simulink model "Model4"  (R2024b)
settings: Solver=VariableStepAuto  StartTime=0.0  StopTime=10.0  RelTol=1e-3
libraries: spsPower3phInstantaneousLib x8, spsThreePhaseParallelRLCLoadLib x4, spsThreePhaseVIMeasurementLib x4, spsThreePhaseBreakerLib x1, spsAsynchronousMachinepuUnitsLib x1, spsExcitationSystemLib x1, spsThreePhaseTransformerTwoWindingsLib x1, spsSynchronousMachinepuStandardLib x1, spsWindTurbineInductionGeneratorPhasorTypeLib x1, spspowerguiLib x1, sps_lib x1
settings Model: Creator=skill  LastModifiedBy=skill

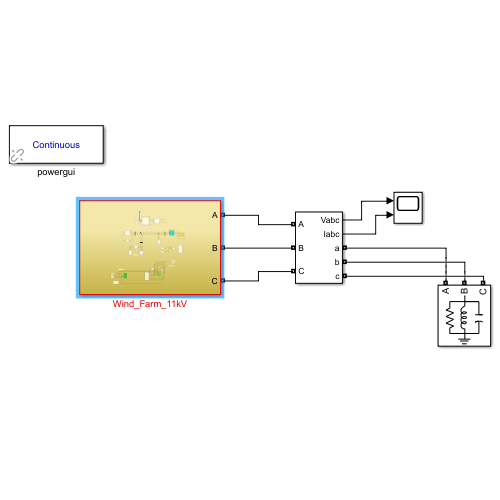
[thumbnail: Simulink's stored preview of the top-level diagram]
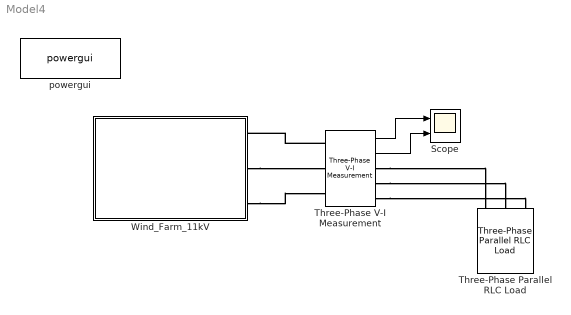
== system Model4 ==
  Scope : Scope  NumInputPorts=2
  Three-Phase Parallel RLC Load : spsThreePhaseParallelRLCLoadLib/Three-Phase Parallel RLC Load  LConnTagsString=A|B|C  Configuration=Y (grounded)  NominalVoltage=1000  Vabc=[1e3 1e3 1e3]  Vabcp=[1e3 1e3 1e3]  NominalFrequency=60  UnbalancedPower=off  ActivePower=10e3  InductivePower=100  CapacitivePower=100  Pabc=[10e3 9e3 11e3]  QLabc=[100 90 110]  QCabc=[100 90 110]  Pabcp=[10e3 9e3 11e3]  QLabcp=[100 90 110]  QCabcp=[100 90 110]  Measurements=None  LoadType=constant Z
  Three-Phase V-I Measurement : spsThreePhaseVIMeasurementLib/Three-Phase V-I Measurement  VoltageMeasurement=phase-to-ground  SetLabelV=off  LabelV=Vabc  Vpu=off  VpuLL=off  CurrentMeasurement=yes  SetLabelI=off  LabelI=Iabc  Ipu=off  Pbase=100e6  Vbase=500e3  OutputType=Complex  PhasorSimulation=off  PSBequivalent=0
  Wind_Farm_11kV : Subsystem
  powergui : sps_lib/powergui  Priority=1  SimulationMode=Continuous  SampleTime=50e-6  frequency=50  Iterations=50  frequencyindice=50  Pbase=100e6  ErrMax=1e-4  UnitsV=kV  UnitsW=MW  buscounter=0  FunctionMessages=off  echomessages=off  EnableUseOfTLC=off  CurrentSourceSwitches=off  DisableSnubberDevices=off  DisableRonSwitches=off  DisableVfSwitches=off  DisplayEquations=off  AutomaticDiscreteSolvers=off  SolverType=Tustin/Backward Euler (TBE)  Interpol=off  ExternalGateDelay=off  methode=off  Ts=100  x0status=blocks  SPID=on  SwTol=0  HookPort=off  NonlinearTolerance=1e-4  nMaxIteration=100  ContinueOnMaxIteration=off  RestoreLinks=warning  ResistiveCurrentMeasurement=off  Frange=[0:2:500]  Ylog=off  Xlog=on  ShowGrid=off  save=off  variable=ZData  structure=0  ZoomFFT=off  StartTime=0.0  cycles=1  DisplayStyle=1  fundamental=60  FreqAxis=off  MaxFrequency=1000  frequencyindicesteady=1  RmsSteady=1  display=off
  wires:
  Three-Phase V-I Measurement/1 -> Scope/1
  Three-Phase V-I Measurement/2 -> Scope/2
  connections:
  Three-Phase V-I Measurement/LConn1 -- Wind_Farm_11kV/RConn1
  Wind_Farm_11kV/RConn2 -- Three-Phase V-I Measurement/LConn2
  Wind_Farm_11kV/RConn3 -- Three-Phase V-I Measurement/LConn3
  Three-Phase V-I Measurement/RConn1 -- Three-Phase Parallel RLC Load/LConn1
  Three-Phase V-I Measurement/RConn2 -- Three-Phase Parallel RLC Load/LConn2
  Three-Phase V-I Measurement/RConn3 -- Three-Phase Parallel RLC Load/LConn3

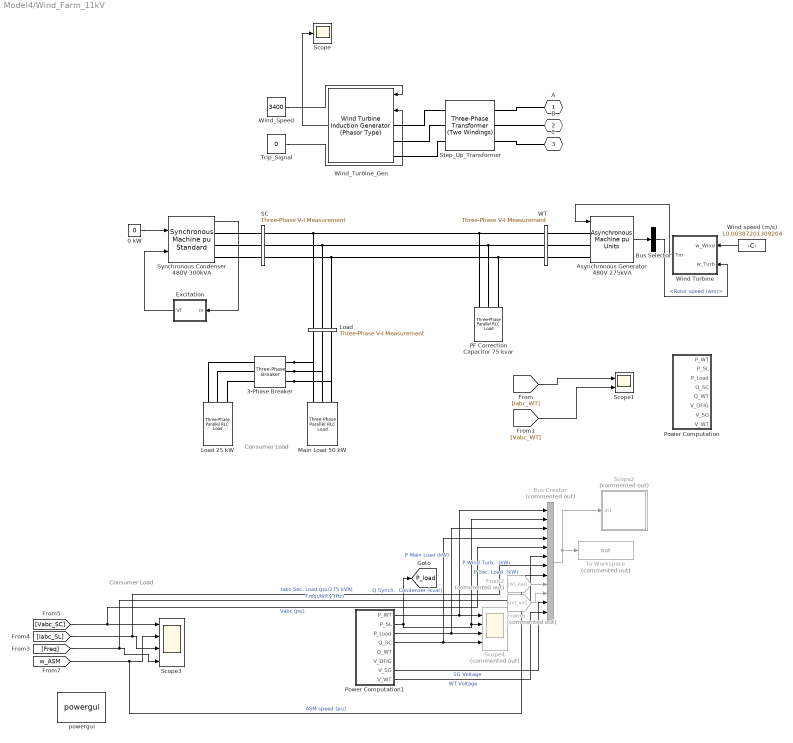
== system Model4/Wind_Farm_11kV ==
  note: Consumer Load
  note: Consumer Load
  0 kW : Constant  Value=0
  3-Phase Breaker : spsThreePhaseBreakerLib/Three-Phase Breaker  InitialState=open  SwitchA=on  SwitchB=on  SwitchC=on  SwitchTimes=[0.2]  External=off  BreakerResistance=0.001  SnubberResistance=1e6  SnubberCapacitance=inf  Measurements=None
      settings: AttributesFormatString=\n
  Asynchronous Generator 480V 275kVA : spsAsynchronousMachinepuUnitsLib/Asynchronous Machine pu Units  RotorType=Squirrel-cage  PresetModel=No  MechanicalLoad=Torque Tm  ShowDetailedParameters=on  ReferenceFrame=Rotor  Units=pu  MeasurementBus=off  NominalParameters=[ 275e3, 480, 60 ]  VoltageRatio=1  Stator=[ 0.016,0.06]  Rotor=[ 0.015,0.06]  Cage1=[0.01909 0.0397]  Cage2=[0.01909 0.0397]  Lm=3.5  Mechanical=[ 2,0,2 ]  PolePairs=2  InitialConditions=[-8.89496e-048 0 0.280896 0.280896 0.280896 -89.7425 150.258 30.2575]  SimulateSaturation=off  Saturation=[ 0 0 ; 0 0 ]  LoadFlowParameters=0  TsPowergui=0  TsBlock=-1  IterativeModel=Trapezoidal non iterative  IterativeDiscreteModel=Trapezoidal non iterative  Pmec=0
      settings: AttributesFormatString=\n
  Bus Creator : BusCreator  Commented=on  Inputs=12
  Bus Selector : BusSelector  OutputSignals=Mechanical.Rotor speed (wm)
  Excitation : Subsystem
  From2 : From  Commented=on  GotoTag=WT_Rea  TagVisibility=global
  From8 : From  Commented=on  GotoTag=rot_vol  TagVisibility=global
  Load : spsThreePhaseVIMeasurementLib/Three-Phase V-I Measurement  VoltageMeasurement=phase-to-ground  SetLabelV=on  LabelV=Vabc_Load  Vpu=on  VpuLL=off  CurrentMeasurement=yes  SetLabelI=on  LabelI=Iabc_Load  Ipu=on  Pbase=275e3  Vbase=480  OutputType=Magnitude  PhasorSimulation=off  PSBequivalent=0
  Load 25 kW : spsThreePhaseParallelRLCLoadLib/Three-Phase Parallel RLC Load  LConnTagsString=A|B|C  Configuration=Y (grounded)  NominalVoltage=480  Vabc=[1e3 1e3 1e3]  Vabcp=[1e3 1e3 1e3]  NominalFrequency=60  UnbalancedPower=off  ActivePower=25e3  InductivePower=0  CapacitivePower=0  Pabc=[10e3 9e3 11e3]  QLabc=[100 90 110]  QCabc=[100 90 110]  Pabcp=[10e3 9e3 11e3]  QLabcp=[100 90 110]  QCabcp=[100 90 110]  Measurements=None  LoadType=constant Z
  Main Load 50 kW : spsThreePhaseParallelRLCLoadLib/Three-Phase Parallel RLC Load  LConnTagsString=A|B|C  Configuration=Y (grounded)  NominalVoltage=480  Vabc=[1e3 1e3 1e3]  Vabcp=[1e3 1e3 1e3]  NominalFrequency=60  UnbalancedPower=off  ActivePower=50e3  InductivePower=0  CapacitivePower=0  Pabc=[10e3 9e3 11e3]  QLabc=[100 90 110]  QCabc=[100 90 110]  Pabcp=[10e3 9e3 11e3]  QLabcp=[100 90 110]  QCabcp=[100 90 110]  Measurements=None  LoadType=constant Z
  PF Correction Capacitor 75 kvar : spsThreePhaseParallelRLCLoadLib/Three-Phase Parallel RLC Load  LConnTagsString=A|B|C  Configuration=Delta  NominalVoltage=480  Vabc=[1e3 1e3 1e3]  Vabcp=[1e3 1e3 1e3]  NominalFrequency=60  UnbalancedPower=off  ActivePower=0  InductivePower=0  CapacitivePower=75e3  Pabc=[10e3 9e3 11e3]  QLabc=[100 90 110]  QCabc=[100 90 110]  Pabcp=[10e3 9e3 11e3]  QLabcp=[100 90 110]  QCabcp=[100 90 110]  Measurements=None  LoadType=constant Z
  Power Computation : Subsystem
  Power Computation1 : Subsystem
  SC : spsThreePhaseVIMeasurementLib/Three-Phase V-I Measurement  VoltageMeasurement=phase-to-ground  SetLabelV=on  LabelV=Vabc_SC  Vpu=on  VpuLL=off  CurrentMeasurement=yes  SetLabelI=on  LabelI=Iabc_SC  Ipu=on  Pbase=300e3  Vbase=480  OutputType=Magnitude  PhasorSimulation=off  PSBequivalent=0
  Scope : Scope
  Scope1 : Scope  NumInputPorts=2
  Scope2 : Subsystem  Commented=on
  Scope3 : Scope  NumInputPorts=4
  Scope4 : Scope  Commented=on  NumInputPorts=4
  Step_Up_Transformer : spsThreePhaseTransformerTwoWindingsLib/Three-Phase Transformer (Two Windings)  Winding1Connection=Yg  Winding2Connection=Yg  CoreType=Three single-phase transformers  SetSaturation=off  Hysteresis=off  DataFile='hysteresis'  SetInitialFlux=off  Measurements=None  UNITS=pu  NominalPower=[2e6, 50]  Winding1=[ 575 , 0.002 , 0.08 ]  Winding2=[ 11e3 , 0.002 , 0.08 ]  Rm=500  Lm=500  L0=0.5  Saturation=[ 0,0 ; 0.0024,1.2 ; 1.0,1.52 ]  InitialFluxes=[ 0.8 , -0.8 , 0.7 ]  BreakLoop=off  DiscreteSolver=Trapezoidal iterative  DataType=off  TransfoNumber=1
  Synchronous Condenser 480V 300kVA : spsSynchronousMachinepuStandardLib/Synchronous Machine pu Standard  PresetModel=No  MechanicalLoad=Mechanical power Pm  ShowDetailedParameters=on  RotorType=Salient-pole  Units=per unit standard parameters  MeasurementBus=off  NominalParameters=[ 300e3 480 60 ]  Reactances1=[ 3.23, 0.21, 0.15, 2.79, 1.03, 0.37, 0.09 ]  Reactances2=[2.24 0.17 0.12 1.02 0.13 0.08]  dAxisTimeConstants=Open-circuit  qAxisTimeConstants=Open-circuit  TimeConstants1="[ 4.4849  0.0681  0.1  ]"  TimeConstants2=[ 1.7, 0.008, 0.213, 0.004 ]  TimeConstants3="[  1.7 0.008 0.051266  ]"  TimeConstants4=[ 8.0, 0.03, 0.3371, 0.0295 ]  TimeConstants5="[ 0.08  0.019  0.004 ]"  TimeConstants6=[ 1.3201, 0.023, 1.0, 0.07 ]  TimeConstants7="[  0.08  0.019 0.051266  ]"  TimeConstants8=[ 1.3201, 0.0231, 0.3371, 0.0295 ]  StatorResistance=0.017  Mechanical=[ 1, 0, 2 ]  PolePairs=2  InitialConditions=[0 -89.2146 0.827 0.827 0.827 -86.4 153.6 33.6 2.71455]  SetSaturation=off  Saturation=[0.6404,0.7127,0.8441,0.9214,0.9956,1.082,1.19,1.316,1.457;0.7,0.7698,0.8872,0.9466,0.9969,1.046,1.1,1.151,1.201]  LoadFlowParameters=[2 0 0 0 0]  TsPowergui=0  TsBlock=-1  IterativeModel=Trapezoidal non iterative  IterativeDiscreteModel=Trapezoidal non iterative  BusType=PV  Pref=0  Qref=0  Qmin=-inf  Qmax=inf  PLF=0  QLF=0
  To Workspace : ToWorkspace  Commented=on  VariableName=out  SaveFormat=Timeseries  SampleTime=-1
  Trip_Signal : Constant  Value=0
  WT : spsThreePhaseVIMeasurementLib/Three-Phase V-I Measurement  VoltageMeasurement=phase-to-ground  SetLabelV=on  LabelV=Vabc_WT  Vpu=on  VpuLL=off  CurrentMeasurement=yes  SetLabelI=on  LabelI=Iabc_WT  Ipu=on  Pbase=275e3  Vbase=480  OutputType=Magnitude  PhasorSimulation=off  PSBequivalent=0
  Wind Turbine : Subsystem
  Wind speed (m/s) : Constant  Value=10.00387201309204
  Wind_Speed : Constant  Value=3400
  Wind_Turbine_Gen : spsWindTurbineInductionGeneratorPhasorTypeLib/Wind Turbine Induction Generator (Phasor Type)  ExternalTm=off  nom=[1.5e6/0.9, 575, 50]  sta=[ 0.004843, 0.1248]  rot=[ 0.004377, 0.1791]  Lm=6.77  mec=[5.04, 0.01, 3]  init="[ -0.01,0,   0,0,0,   0,0,0 ]"  pitch_angle=0  Pmec=1.5e6  wind_base=9  speed_nom=1  P_wind_base=1  K_pitch_gain=[5 25]  pitch_max=45  pitch_rate=2
      settings: LibrarySourceBlock=|
      | sps_lib/Electrical Machines/Wind Turbine
      | Induction Generator
      | (Phasor Type)
  powergui : spspowerguiLib/powergui  SimulationMode=Continuous  SampleTime=0  frequency=60  Iterations=50  frequencyindice=60  Pbase=100e6  ErrMax=1e-4  UnitsV=kV  UnitsW=MW  buscounter=0  FunctionMessages=off  echomessages=off  EnableUseOfTLC=off  CurrentSourceSwitches=on  DisableSnubberDevices=on  DisableRonSwitches=off  DisableVfSwitches=off  DisplayEquations=off  AutomaticDiscreteSolvers=off  SolverType=Tustin  Interpol=off  ExternalGateDelay=off  methode=off  Ts=0  x0status=blocks  SPID=off  SwTol=0  HookPort=off  NonlinearTolerance=1e-4  nMaxIteration=100  ContinueOnMaxIteration=off  RestoreLinks=warning  ResistiveCurrentMeasurement=off  Frange=[0:2:500]  Ylog=off  Xlog=on  ShowGrid=off  save=off  variable=ZData  structure=0  ZoomFFT=on  StartTime=0.0  cycles=1  DisplayStyle=1  fundamental=60  FreqAxis=off  MaxFrequency=1000  frequencyindicesteady=1  RmsSteady=1  display=off
  A : PMIOPort  Side=Right
  B : PMIOPort  Port=2  Side=Right
  C : PMIOPort  Port=3  Side=Right
  tag scope: P_load=global
  wires:
  Wind_Speed/1 -> Wind_Turbine_Gen/1
  Trip_Signal/1 -> Wind_Turbine_Gen/2
  Wind_Turbine_Gen/1 -> Scope/1
  Wind speed (m/s)/1 -> Wind Turbine/1(w_Wind)
  Asynchronous Generator 480V 275kVA/1 -> Bus Selector/1
  Bus Selector/1 -> Wind Turbine/2(w_Turb)  "<Rotor speed (wm)>"
  Wind Turbine/1(Tm) -> Asynchronous Generator 480V 275kVA/1
  Synchronous Condenser 480V 300kVA/1 -> Excitation/1(m)
  Excitation/1(Vf) -> Synchronous Condenser 480V 300kVA/2
  0 kW/1 -> Synchronous Condenser 480V 300kVA/1
  [Iabc_WT] -> Scope1/1
  [Vabc_WT] -> Scope1/2
  Power Computation1/1(P_WT) -> Bus Creator/1, Scope4/1  "P Wind Turb.  (kW)"
  Power Computation1/2(P_SL) -> Bus Creator/2, Scope4/2, [P_load]  "P Sec. Load  (kW)"
  Power Computation1/7(V_SG) -> Bus Creator/11  "SG Voltage"
  [Vabc_SC] -> Bus Creator/5, Scope3/1  "Vabc (pu)"
  Bus Creator/1 -> Scope2/1(In1), To Workspace/1
  [Iabc_SL] -> Bus Creator/7, Scope3/3  "Iabc Sec. Load (pu/275 kVA)"
  Power Computation1/3(P_Load) -> Bus Creator/3, Scope4/3  "P Main Load (kW)"
  Power Computation1/4(Q_SC) -> Bus Creator/4, Scope4/4  "Q Synch.  Condenser (kvar)"
  From8/1 -> Bus Creator/10
  [w_ASM] -> Bus Creator/8, Scope3/2  "ASM speed (pu)"
  From2/1 -> Bus Creator/9
  [Freq] -> Bus Creator/6, Scope3/4  "Frequency (Hz)"
  Power Computation1/8(V_WT) -> Bus Creator/12  "WT Voltage"
  connections:
  Wind_Turbine_Gen/LConn1 -- Step_Up_Transformer/LConn1
  Wind_Turbine_Gen/LConn2 -- Step_Up_Transformer/LConn2
  Wind_Turbine_Gen/LConn3 -- Step_Up_Transformer/LConn3
  Step_Up_Transformer/RConn1 -- A/RConn1
  Step_Up_Transformer/RConn2 -- B/RConn1
  Step_Up_Transformer/RConn3 -- C/RConn1
  WT/RConn1 -- Asynchronous Generator 480V 275kVA/LConn1
  WT/RConn2 -- Asynchronous Generator 480V 275kVA/LConn2
  WT/RConn3 -- Asynchronous Generator 480V 275kVA/LConn3
  SC/RConn1 -- Load/LConn1 -- PF Correction Capacitor 75 kvar/LConn1 -- WT/LConn1
  SC/RConn2 -- Load/LConn2 -- WT/LConn2 -- PF Correction Capacitor 75 kvar/LConn2
  SC/RConn3 -- Load/LConn3 -- PF Correction Capacitor 75 kvar/LConn3 -- WT/LConn3
  Synchronous Condenser 480V 300kVA/RConn1 -- SC/LConn1
  Synchronous Condenser 480V 300kVA/RConn2 -- SC/LConn2
  Synchronous Condenser 480V 300kVA/RConn3 -- SC/LConn3
  3-Phase Breaker/LConn2 -- Load/RConn2 -- Main Load 50 kW/LConn2
  3-Phase Breaker/LConn1 -- Load/RConn1 -- Main Load 50 kW/LConn1
  3-Phase Breaker/LConn3 -- Load/RConn3 -- Main Load 50 kW/LConn3
  3-Phase Breaker/RConn2 -- Load 25 kW/LConn2
  3-Phase Breaker/RConn1 -- Load 25 kW/LConn1
  3-Phase Breaker/RConn3 -- Load 25 kW/LConn3

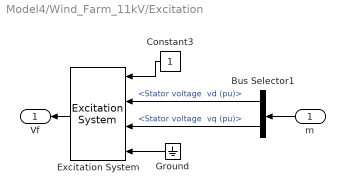
== system Model4/Wind_Farm_11kV/Excitation ==
  m : Inport
  Bus Selector1 : BusSelector  OutputSignals="dq0 components.Stator voltage  vd (pu),dq0 components.Stator voltage  vq (pu)"
  Constant3 : Constant
  Excitation System : spsExcitationSystemLib/Excitation System  tr=20e-3  reg=[ 300, 0.001 ]  exc=[ 1, 0 ]  tgr=[ 0, 0 ]  damp=[ 0.001, 0.1 ]  sat=[ 0, 0 ]  lim=[ -11.5, 11.5, 0 ]  v0=[1,2.71455]
  Ground : Ground
  Vf : Outport  VectorParamsAs1DForOutWhenUnconnected=off
  wires:
  Constant3/1 -> Excitation System/1
  Ground/1 -> Excitation System/4
  m/1 -> Bus Selector1/1
  Excitation System/1 -> Vf/1
  Bus Selector1/1 -> Excitation System/2  "<Stator voltage  vd (pu)>"
  Bus Selector1/2 -> Excitation System/3  "<Stator voltage  vq (pu)>"

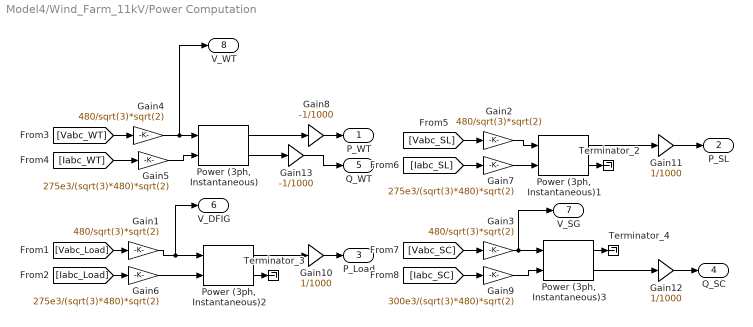
== system Model4/Wind_Farm_11kV/Power Computation ==
  Gain{1..4} (4 alike) : Gain  Gain=480/sqrt(3)*sqrt(2)  SaturateOnIntegerOverflow=on  OutDataTypeStr=Inherit: Same as input  ParamDataTypeStr=Inherit: Same as input
  Gain10 : Gain  Gain=1/1000  SaturateOnIntegerOverflow=on  OutDataTypeStr=Inherit: Same as input  ParamDataTypeStr=Inherit: Same as input
  Gain11 : Gain  Gain=1/1000  SaturateOnIntegerOverflow=on  OutDataTypeStr=Inherit: Same as input  ParamDataTypeStr=Inherit: Same as input
  Gain12 : Gain  Gain=1/1000  SaturateOnIntegerOverflow=on  OutDataTypeStr=Inherit: Same as input  ParamDataTypeStr=Inherit: Same as input
  Gain13 : Gain  Gain=-1/1000  SaturateOnIntegerOverflow=on  OutDataTypeStr=Inherit: Same as input  ParamDataTypeStr=Inherit: Same as input
  Gain5 : Gain  Gain=275e3/(sqrt(3)*480)*sqrt(2)  SaturateOnIntegerOverflow=on  OutDataTypeStr=Inherit: Same as input  ParamDataTypeStr=Inherit: Same as input
  Gain6 : Gain  Gain=275e3/(sqrt(3)*480)*sqrt(2)  SaturateOnIntegerOverflow=on  OutDataTypeStr=Inherit: Same as input  ParamDataTypeStr=Inherit: Same as input
  Gain7 : Gain  Gain=275e3/(sqrt(3)*480)*sqrt(2)  SaturateOnIntegerOverflow=on  OutDataTypeStr=Inherit: Same as input  ParamDataTypeStr=Inherit: Same as input
  Gain8 : Gain  Gain=-1/1000  SaturateOnIntegerOverflow=on  OutDataTypeStr=Inherit: Same as input  ParamDataTypeStr=Inherit: Same as input
  Gain9 : Gain  Gain=300e3/(sqrt(3)*480)*sqrt(2)  SaturateOnIntegerOverflow=on  OutDataTypeStr=Inherit: Same as input  ParamDataTypeStr=Inherit: Same as input
  Power (3ph, Instantaneous){,1..3} (4 alike) : spsPower3phInstantaneousLib/Power (3ph, Instantaneous)
  Terminator_2 : Terminator
  Terminator_3 : Terminator
  Terminator_4 : Terminator
  P_WT : Outport  VectorParamsAs1DForOutWhenUnconnected=off
  P_SL : Outport  Port=2  VectorParamsAs1DForOutWhenUnconnected=off
  P_Load : Outport  Port=3  VectorParamsAs1DForOutWhenUnconnected=off
  Q_SC : Outport  Port=4  VectorParamsAs1DForOutWhenUnconnected=off
  Q_WT : Outport  Port=5  VectorParamsAs1DForOutWhenUnconnected=off
  V_DFIG : Outport  Port=6  VectorParamsAs1DForOutWhenUnconnected=off
  V_SG : Outport  Port=7  VectorParamsAs1DForOutWhenUnconnected=off
  V_WT : Outport  Port=8  VectorParamsAs1DForOutWhenUnconnected=off
  wires:
  "Power (3ph, Instantaneous)1"/1 -> Gain11/1
  [Vabc_WT] -> Gain4/1
  [Iabc_WT] -> Gain5/1
  Gain4/1 -> V_WT/1, "Power (3ph, Instantaneous)"/1
  Gain5/1 -> "Power (3ph, Instantaneous)"/2
  [Vabc_Load] -> Gain1/1
  [Iabc_Load] -> Gain6/1
  Gain1/1 -> V_DFIG/1, "Power (3ph, Instantaneous)2"/1
  Gain6/1 -> "Power (3ph, Instantaneous)2"/2
  [Vabc_SL] -> Gain2/1
  [Iabc_SL] -> Gain7/1
  Gain2/1 -> "Power (3ph, Instantaneous)1"/1
  Gain7/1 -> "Power (3ph, Instantaneous)1"/2
  "Power (3ph, Instantaneous)2"/1 -> Gain10/1
  "Power (3ph, Instantaneous)"/1 -> Gain8/1
  Gain8/1 -> P_WT/1
  "Power (3ph, Instantaneous)3"/2 -> Gain12/1
  [Vabc_SC] -> Gain3/1
  [Iabc_SC] -> Gain9/1
  Gain3/1 -> V_SG/1, "Power (3ph, Instantaneous)3"/1
  Gain9/1 -> "Power (3ph, Instantaneous)3"/2
  Gain10/1 -> P_Load/1
  Gain11/1 -> P_SL/1
  Gain12/1 -> Q_SC/1
  "Power (3ph, Instantaneous)"/2 -> Gain13/1
  "Power (3ph, Instantaneous)1"/2 -> Terminator_2/1
  "Power (3ph, Instantaneous)2"/2 -> Terminator_3/1
  "Power (3ph, Instantaneous)3"/1 -> Terminator_4/1
  Gain13/1 -> Q_WT/1

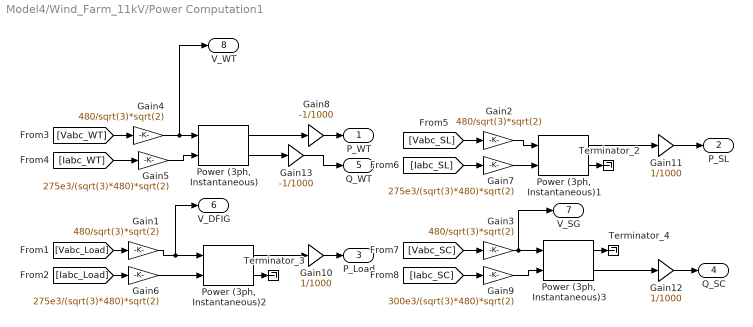
== system Model4/Wind_Farm_11kV/Power Computation1 ==
  Gain{1..4} (4 alike) : Gain  Gain=480/sqrt(3)*sqrt(2)  SaturateOnIntegerOverflow=on  OutDataTypeStr=Inherit: Same as input  ParamDataTypeStr=Inherit: Same as input
  Gain10 : Gain  Gain=1/1000  SaturateOnIntegerOverflow=on  OutDataTypeStr=Inherit: Same as input  ParamDataTypeStr=Inherit: Same as input
  Gain11 : Gain  Gain=1/1000  SaturateOnIntegerOverflow=on  OutDataTypeStr=Inherit: Same as input  ParamDataTypeStr=Inherit: Same as input
  Gain12 : Gain  Gain=1/1000  SaturateOnIntegerOverflow=on  OutDataTypeStr=Inherit: Same as input  ParamDataTypeStr=Inherit: Same as input
  Gain13 : Gain  Gain=-1/1000  SaturateOnIntegerOverflow=on  OutDataTypeStr=Inherit: Same as input  ParamDataTypeStr=Inherit: Same as input
  Gain5 : Gain  Gain=275e3/(sqrt(3)*480)*sqrt(2)  SaturateOnIntegerOverflow=on  OutDataTypeStr=Inherit: Same as input  ParamDataTypeStr=Inherit: Same as input
  Gain6 : Gain  Gain=275e3/(sqrt(3)*480)*sqrt(2)  SaturateOnIntegerOverflow=on  OutDataTypeStr=Inherit: Same as input  ParamDataTypeStr=Inherit: Same as input
  Gain7 : Gain  Gain=275e3/(sqrt(3)*480)*sqrt(2)  SaturateOnIntegerOverflow=on  OutDataTypeStr=Inherit: Same as input  ParamDataTypeStr=Inherit: Same as input
  Gain8 : Gain  Gain=-1/1000  SaturateOnIntegerOverflow=on  OutDataTypeStr=Inherit: Same as input  ParamDataTypeStr=Inherit: Same as input
  Gain9 : Gain  Gain=300e3/(sqrt(3)*480)*sqrt(2)  SaturateOnIntegerOverflow=on  OutDataTypeStr=Inherit: Same as input  ParamDataTypeStr=Inherit: Same as input
  Power (3ph, Instantaneous){,1..3} (4 alike) : spsPower3phInstantaneousLib/Power (3ph, Instantaneous)
  Terminator_2 : Terminator
  Terminator_3 : Terminator
  Terminator_4 : Terminator
  P_WT : Outport  VectorParamsAs1DForOutWhenUnconnected=off
  P_SL : Outport  Port=2  VectorParamsAs1DForOutWhenUnconnected=off
  P_Load : Outport  Port=3  VectorParamsAs1DForOutWhenUnconnected=off
  Q_SC : Outport  Port=4  VectorParamsAs1DForOutWhenUnconnected=off
  Q_WT : Outport  Port=5  VectorParamsAs1DForOutWhenUnconnected=off
  V_DFIG : Outport  Port=6  VectorParamsAs1DForOutWhenUnconnected=off
  V_SG : Outport  Port=7  VectorParamsAs1DForOutWhenUnconnected=off
  V_WT : Outport  Port=8  VectorParamsAs1DForOutWhenUnconnected=off
  wires:
  "Power (3ph, Instantaneous)1"/1 -> Gain11/1
  [Vabc_WT] -> Gain4/1
  [Iabc_WT] -> Gain5/1
  Gain4/1 -> V_WT/1, "Power (3ph, Instantaneous)"/1
  Gain5/1 -> "Power (3ph, Instantaneous)"/2
  [Vabc_Load] -> Gain1/1
  [Iabc_Load] -> Gain6/1
  Gain1/1 -> V_DFIG/1, "Power (3ph, Instantaneous)2"/1
  Gain6/1 -> "Power (3ph, Instantaneous)2"/2
  [Vabc_SL] -> Gain2/1
  [Iabc_SL] -> Gain7/1
  Gain2/1 -> "Power (3ph, Instantaneous)1"/1
  Gain7/1 -> "Power (3ph, Instantaneous)1"/2
  "Power (3ph, Instantaneous)2"/1 -> Gain10/1
  "Power (3ph, Instantaneous)"/1 -> Gain8/1
  Gain8/1 -> P_WT/1
  "Power (3ph, Instantaneous)3"/2 -> Gain12/1
  [Vabc_SC] -> Gain3/1
  [Iabc_SC] -> Gain9/1
  Gain3/1 -> V_SG/1, "Power (3ph, Instantaneous)3"/1
  Gain9/1 -> "Power (3ph, Instantaneous)3"/2
  Gain10/1 -> P_Load/1
  Gain11/1 -> P_SL/1
  Gain12/1 -> Q_SC/1
  "Power (3ph, Instantaneous)"/2 -> Gain13/1
  "Power (3ph, Instantaneous)1"/2 -> Terminator_2/1
  "Power (3ph, Instantaneous)2"/2 -> Terminator_3/1
  "Power (3ph, Instantaneous)3"/1 -> Terminator_4/1
  Gain13/1 -> Q_WT/1

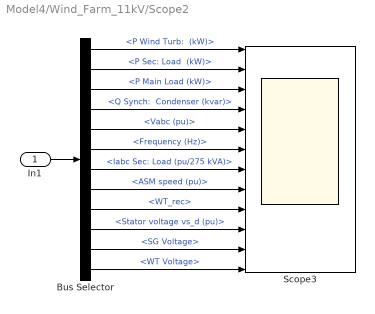
== system Model4/Wind_Farm_11kV/Scope2 ==
  In1 : Inport
  Bus Selector : BusSelector  OutputSignals="P Wind Turb:  (kW),P Sec: Load  (kW),P Main Load (kW),Q Synch:  Condenser (kvar),Vabc (pu),Frequency (Hz),Iabc Sec: Load (pu/275 kVA),ASM speed (pu),WT_rec,Stator voltage vs_d (pu),SG Voltage,WT Voltage"
  Scope3 : Scope  NumInputPorts=12
  wires:
  In1/1 -> Bus Selector/1
  Bus Selector/1 -> Scope3/1  "<P Wind Turb:  (kW)>"
  Bus Selector/2 -> Scope3/2  "<P Sec: Load  (kW)>"
  Bus Selector/3 -> Scope3/3  "<P Main Load (kW)>"
  Bus Selector/4 -> Scope3/4  "<Q Synch:  Condenser (kvar)>"
  Bus Selector/5 -> Scope3/5  "<Vabc (pu)>"
  Bus Selector/6 -> Scope3/6  "<Frequency (Hz)>"
  Bus Selector/7 -> Scope3/7  "<Iabc Sec: Load (pu/275 kVA)>"
  Bus Selector/8 -> Scope3/8  "<ASM speed (pu)>"
  Bus Selector/9 -> Scope3/9  "<WT_rec>"
  Bus Selector/10 -> Scope3/10  "<Stator voltage vs_d (pu)>"
  Bus Selector/11 -> Scope3/11  "<SG Voltage>"
  Bus Selector/12 -> Scope3/12  "<WT Voltage>"

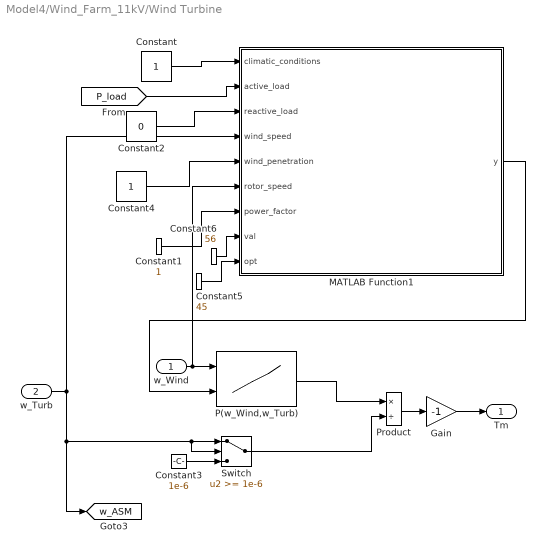
== system Model4/Wind_Farm_11kV/Wind Turbine ==
  w_Wind : Inport
  w_Turb : Inport  Port=2
  Constant : Constant
  Constant1 : Constant
  Constant2 : Constant  Value=0
  Constant3 : Constant  Value=1e-6
  Constant4 : Constant
  Constant5 : Constant  Value=45
  Constant6 : Constant  Value=56
  Gain : Gain  Gain=-1  SaturateOnIntegerOverflow=on  OutDataTypeStr=Inherit: Same as input  ParamDataTypeStr=Inherit: Same as input
  MATLAB Function1 : MATLAB Function  TreatAsAtomicUnit=on
  P(w_Wind,w_Turb) : Lookup_n-D  BreakpointsForDimension1=[0 5 6 7 8 9 10 11 12]  BreakpointsForDimension2=[0 571.55 685.8 800.15 914.4 1028.8 1143.1 1257.4 1371.7 1486 1600.3 1714.6 1828.9 1943.2 2057.5 2171.8 2286.1 2400.5 2514.7 2629.1 2743.3 2857.7 2971.9 3086.3 3200.5 3314.9 3429.2]  Table=[0 5 6 7 8 9 10 11 12]  InternalRulePriority=Speed  RndMeth=Simplest
      settings: InputPortMap=u0,u1
  Product : Product  Inputs=*/  InputSameDT=on  SaturateOnIntegerOverflow=on  OutDataTypeStr=Inherit: Same as first input
  Switch : Switch  Threshold=1e-6
  Tm : Outport  VectorParamsAs1DForOutWhenUnconnected=off
  tag scope: w_ASM=global
  wires:
  Constant3/1 -> Switch/3
  w_Wind/1 -> MATLAB Function1/6(rotor_speed), P(w_Wind,w_Turb)/1
  P(w_Wind,w_Turb)/1 -> Product/1
  Switch/1 -> Product/2
  Product/1 -> Gain/1
  Gain/1 -> Tm/1
  [P_load] -> MATLAB Function1/2(active_load)
  Constant1/1 -> MATLAB Function1/7(power_factor)
  Constant2/1 -> MATLAB Function1/3(reactive_load)
  Constant/1 -> MATLAB Function1/1(climatic_conditions)
  Constant4/1 -> MATLAB Function1/5(wind_penetration)
  w_Turb/1 -> MATLAB Function1/4(wind_speed), Switch/1, Switch/2, [w_ASM]
  MATLAB Function1/1(y) -> P(w_Wind,w_Turb)/2
  Constant5/1 -> MATLAB Function1/9(opt)
  Constant6/1 -> MATLAB Function1/8(val)

== matlab function Model4/Wind_Farm_11kV/Wind Turbine/MATLAB Function1 ==
  data: climatic_conditions input; y output; active_load input; reactive_load input; wind_speed input; wind_penetration input; rotor_speed input; power_factor input; val input; opt input
function y = fcn(climatic_conditions, active_load, reactive_load, wind_speed, wind_penetration, rotor_speed, power_factor, val, opt)
    u=[climatic_conditions, active_load, reactive_load, wind_speed, wind_penetration, rotor_speed, power_factor];
    X_train=reshape(u, [ 1, 1, size(u, 2), size(u,1)]);
%     coder.extrinsic('evalin', 'assignin')
%     net = 0;                  % Needed in order to set variable class correctly
%     net = evalin('base','net'); % Read value from workspace
%      net = coder.loadDeepLearningNetwork('DeepNN.mat', 'net'); 
%     y = double(predict(net, X_train));
%     y = double(net.predict(X_train));
    y = 1800 +val(opt);
% y = val;
end
